simulink model "Test_Hardware"  (R2024a)
settings: Solver=FixedStepAuto  StartTime=0.0  StopTime=inf  FixedStep=0.001  RelTol=1e-3  EnableMultiTasking=on
undefined symbols (not defined in the file or in its folder): g, Jr, k, kp, kv, Lr, mr
libraries: arduinolib x3, arduinosensorlib x2, eeGeneralControl x2
settings Model: ExtModeTrigDuration=2  Creator=Ingy  LastModifiedBy=Ingy
settings SolverCC: AutoInsertRateTranBlk=on
settings OptimizationCC: EnhancedBackFolding=on  PassReuseOutputArgsAs=Individual arguments  ZeroExternalMemoryAtStartup=off  ZeroInternalMemoryAtStartup=off  MaxStackSize=64  OptimizeBlockOrder=speed  DifferentSizesBufferReuse=on  OptimizationCustomize=off  EfficientTunableParamExpr=on
settings DebuggingCC: ParameterTunabilityLossMsg=error
settings HardwareCC: ProdBitPerPointer=32  ProdBitPerSizeT=32  ProdBitPerPtrDiffT=32  ProdLargestAtomicInteger=Long  ProdLargestAtomicFloat=Double  ProdWordSize=32  ProdHWDeviceType=ARM Compatible->ARM Cortex  UseEmbeddedCoderFeatures=off
settings SFSimCC: MATLABDynamicMemAlloc=off
settings RTWCC: Description=Embedded Coder  SystemTargetFile=ert.tlc  HardwareBoard=ESP32-WROOM(Arduino Compatible)  TLCOptions="-aInlineSetEventsForThisBaseRateFcn=TLC_FALSE -aSuppressMultiTaskScheduler=TLC_FALSE  -aRateBasedStepFcn=0"  TemplateMakefile=ert_default_tmf  Toolchain=ESP32  BuildConfiguration=Faster Runs
settings CodeAppCC: ForceParamTrailComments=on  IgnoreCustomStorageClasses=off  OperatorAnnotations=on  SimulinkDataObjDesc=on  SFDataObjDesc=on  InsertBlockDesc=on
settings ERTTargetCC: SupportContinuousTime=on  SupportNonInlinedSFcns=on  SupportVariableSizeSignals=on  ExtModeTransport=3  ExtModeStaticAlloc=on  ExtModeAutomaticAllocSize=off  ExtModeStaticAllocSize=65536  ExtModeMexFile=ext_xcp  ExtModeIntrfLevel=Level2 - Open

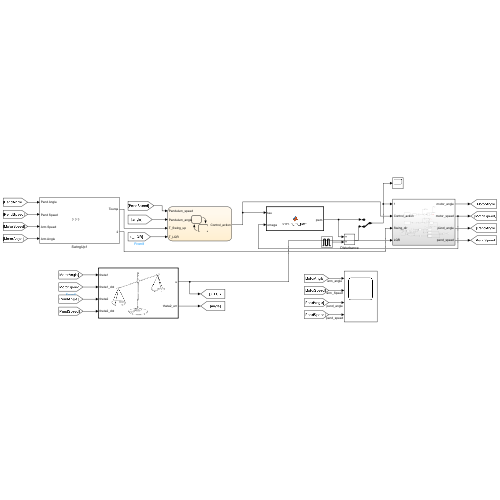
[thumbnail: Simulink's stored preview of the top-level diagram]
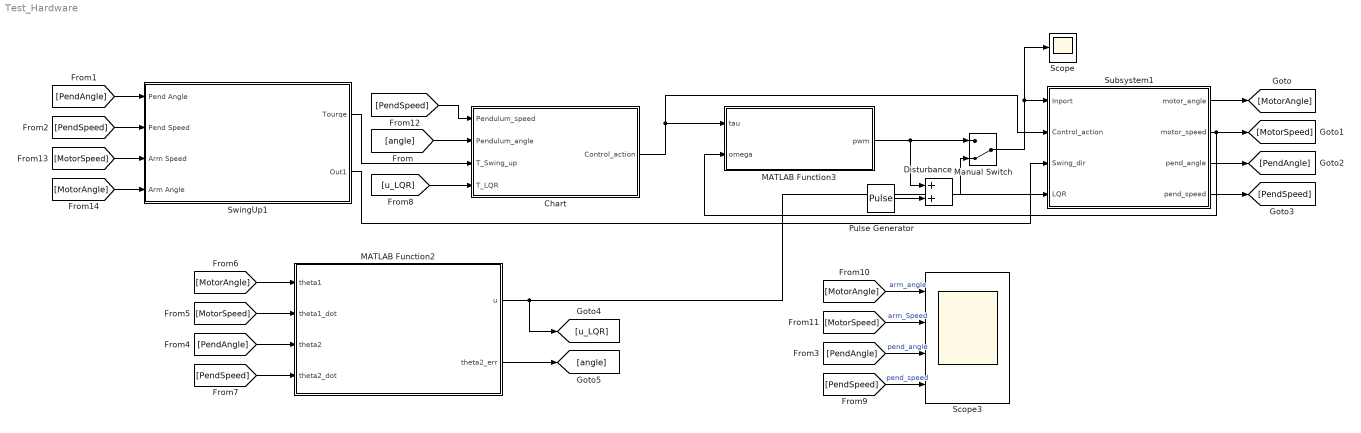
== system Test_Hardware ==
  Chart : Stateflow chart  TreatAsAtomicUnit=on
  Disturbance : Sum
  MATLAB Function2 : MATLAB Function  TreatAsAtomicUnit=on  SystemSampleTime=0.001
  MATLAB Function3 : MATLAB Function  TreatAsAtomicUnit=on
  Manual Switch : ManualSwitch  CurrentSetting=0
  Pulse Generator : DiscretePulseGenerator  PulseType=Time based  Amplitude=90  Period=500  PulseWidth=0.05  PhaseDelay=1
  Scope : Scope
  Scope3 : Scope  NumInputPorts=4
  Subsystem1 : Subsystem
  SwingUp1 : Subsystem
      mask Display: image('download.jpg', [5,5,5,5,100,100]);
  wires:
  [PendAngle] -> SwingUp1/1(Pend Angle)
  Subsystem1/3(pend_angle) -> [PendAngle]
  [PendSpeed] -> Scope3/4  "pend_speed"
  [PendSpeed] -> SwingUp1/2(Pend Speed)
  Subsystem1/1(motor_angle) -> [MotorAngle]
  Subsystem1/4(pend_speed) -> [PendSpeed]
  [MotorAngle] -> Scope3/1  "arm_angle"
  [u_LQR] -> Chart/4(T_LQR)
  [PendAngle] -> Scope3/3  "pend_angle"
  [MotorSpeed] -> Scope3/2  "arm_Speed"
  Manual Switch/1 -> Scope/1, Subsystem1/1(Inport)
  Subsystem1/2(motor_speed) -> MATLAB Function3/2(omega), [MotorSpeed]
  [MotorSpeed] -> SwingUp1/3(Arm Speed)
  [MotorAngle] -> SwingUp1/4(Arm Angle)
  [MotorAngle] -> MATLAB Function2/1(theta1)
  [MotorSpeed] -> MATLAB Function2/2(theta1_dot)
  [PendAngle] -> MATLAB Function2/3(theta2)
  [PendSpeed] -> MATLAB Function2/4(theta2_dot)
  SwingUp1/2(Out1) -> Subsystem1/3(Swing_dir)
  MATLAB Function2/1(u) -> [u_LQR], Subsystem1/4(LQR)
  SwingUp1/1(Tourqe) -> Chart/3(T_Swing_up)
  Chart/1(Control_action) -> Subsystem1/2(Control_action), MATLAB Function3/1(tau)
  MATLAB Function2/2(theta2_err) -> [angle]
  [angle] -> Chart/2(Pendulum_angle)
  [PendSpeed] -> Chart/1(Pendulum_speed)
  Disturbance/1 -> Manual Switch/2
  Pulse Generator/1 -> Disturbance/2
  MATLAB Function3/1(pwm) -> Manual Switch/1, Disturbance/1

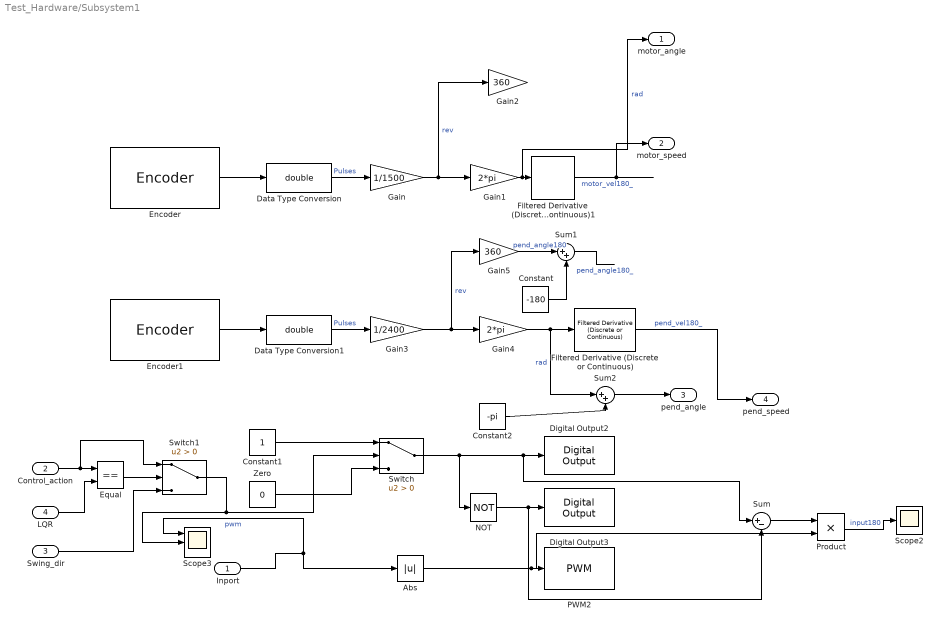
== system Test_Hardware/Subsystem1 ==
  Inport : Inport
  Control_action : Inport  Port=2
  Swing_dir : Inport  Port=3
  LQR : Inport  Port=4
  Abs : Abs  SaturateOnIntegerOverflow=off
  Constant : Constant  Value=-180
  Constant1 : Constant
  Constant2 : Constant  Value=-pi
  Data Type Conversion : DataTypeConversion  OutDataTypeStr=double  SaturateOnIntegerOverflow=off  RndMeth=Floor
  Data Type Conversion1 : DataTypeConversion  OutDataTypeStr=double  SaturateOnIntegerOverflow=off  RndMeth=Floor
  Digital Output2 : arduinolib/Digital Output  pinNumber=23  Direction=output  blockPlatform=arduino
  Digital Output3 : arduinolib/Digital Output  pinNumber=22  Direction=output  blockPlatform=arduino
  Encoder : arduinosensorlib/Encoder  InputA=25  InputB=26  Mode=No reset  SampleTime=-1
  Encoder1 : arduinosensorlib/Encoder  InputA=19  InputB=18  Mode=No reset  SampleTime=-1
  Equal : RelationalOperator  Operator===  OutDataTypeStr=boolean  RndMeth=Simplest  InputSameDT=off
  Filtered Derivative (Discrete or Continuous) : eeGeneralControl/Filtered Derivative (Discrete or Continuous)  K=1  T=0.07  B=inf  A=-inf  minRatio=10  init_option=Inherited from block input  x0=0  Ts=-1
      settings: LibrarySourceBlock=|
      | ee_sl_lib/General Control/Filtered Derivative
      | (Discrete or Continuous)
  Filtered Derivative (Discrete or Continuous)1 : eeGeneralControl/Filtered Derivative (Discrete or Continuous)  K=1  T=0.07  B=inf  A=-inf  minRatio=10  init_option=Inherited from block input  x0=0  Ts=-1
      settings: LibrarySourceBlock=|
      | ee_sl_lib/General Control/Filtered Derivative
      | (Discrete or Continuous)
  Gain : Gain  Gain=1/1500
  Gain1 : Gain  Gain=2*pi
  Gain2 : Gain  Gain=360
  Gain3 : Gain  Gain=1/2400
  Gain4 : Gain  Gain=2*pi
  Gain5 : Gain  Gain=360
  NOT : Logic  Operator=NOT  IconShape=distinctive  AllPortsSameDT=off  OutDataTypeStr=boolean
  PWM2 : arduinolib/PWM  pinNumber=21  frequencyType=Default  desiredFrequency=800  achievableFrequency=800
  Product : Product
  Scope2 : Scope
  Scope3 : Scope  NumInputPorts=3
  Sum : Sum  Inputs=|+-
  Sum1 : Sum  Inputs=|++
  Sum2 : Sum  Inputs=|++
  Switch : Switch  Criteria=u2 > Threshold  SaturateOnIntegerOverflow=off  InputSameDT=off
  Switch1 : Switch  Criteria=u2 > Threshold  SaturateOnIntegerOverflow=off  InputSameDT=off
  Zero : Constant  Value=0  OutDataTypeStr=Inherit: Inherit via back propagation
  motor_angle : Outport
  motor_speed : Outport  Port=2
  pend_angle : Outport  Port=3
  pend_speed : Outport  Port=4
  wires:
  Sum1/1 -> ?  "pend_angle180_"
  Gain5/1 -> Sum1/1  "pend_angle180"
  Filtered Derivative (Discrete or Continuous)1/1 -> motor_speed/1  "motor_vel180_"
  Data Type Conversion/1 -> Gain/1  "Pulses"
  Gain/1 -> Gain2/1, Gain1/1  "rev"
  Filtered Derivative (Discrete or Continuous)/1 -> pend_speed/1  "pend_vel180_"
  Gain4/1 -> Sum2/1, Filtered Derivative (Discrete or Continuous)/1  "rad"
  Data Type Conversion1/1 -> Gain3/1  "Pulses"
  Gain3/1 -> Gain5/1, Gain4/1  "rev"
  Constant/1 -> Sum1/2
  Encoder/1 -> Data Type Conversion/1
  Gain1/1 -> motor_angle/1, Filtered Derivative (Discrete or Continuous)1/1  "rad"
  Encoder1/1 -> Data Type Conversion1/1
  Inport/1 -> Abs/1, Scope3/1  "pwm"
  Constant1/1 -> Switch/1
  Zero/1 -> Switch/3
  NOT/1 -> Sum/2, Digital Output3/1
  Abs/1 -> Product/2, PWM2/1
  Product/1 -> Scope2/1  "input180"
  Sum/1 -> Product/1
  Switch/1 -> NOT/1, Sum/1, Digital Output2/1
  Constant2/1 -> Sum2/2
  Sum2/1 -> pend_angle/1
  LQR/1 -> Equal/2
  Swing_dir/1 -> Switch1/3
  Switch1/1 -> Scope3/2, Switch/2
  Control_action/1 -> Switch1/1, Equal/1
  Equal/1 -> Switch1/2

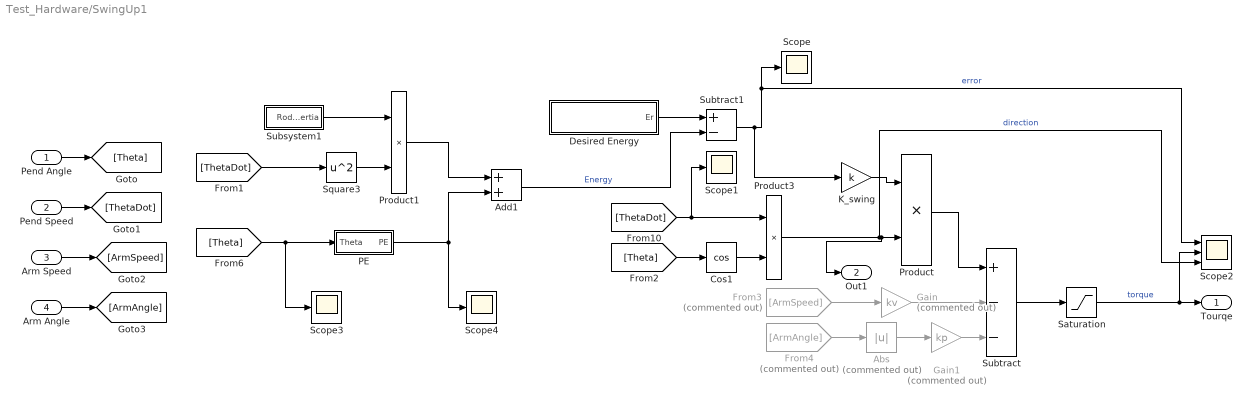
== system Test_Hardware/SwingUp1 ==
  Pend Angle : Inport
  Pend Speed : Inport  Port=2
  Arm Speed : Inport  Port=3
  Arm Angle : Inport  Port=4
  Abs : Abs  Commented=on  SaturateOnIntegerOverflow=off
  Add1 : Sum
  Cos1 : Trigonometry  Operator=cos
  Desired Energy : Subsystem
  From3 : From  Commented=on  GotoTag=ArmSpeed
  From4 : From  Commented=on  GotoTag=ArmAngle
  Gain : Gain  Commented=on  Gain=kv
  Gain1 : Gain  Commented=on  Gain=kp
  K_swing : Gain  Gain=k
  PE : Subsystem
  Product : Product
  Product1 : Product
  Product3 : Product
  Saturation : Saturate  UpperLimit=3  LowerLimit=-3
  Scope{,1,3..4} (4 alike) : Scope
  Scope2 : Scope  NumInputPorts=3
  Square3 : Math  Operator=square
  Subsystem1 : Subsystem
  Subtract : Sum  Inputs=+--
  Subtract1 : Sum  Inputs=+-
  Tourqe : Outport
  Out1 : Outport  Port=2
  wires:
  Pend Angle/1 -> [Theta]
  Pend Speed/1 -> [ThetaDot]
  Subsystem1/1(RodInertia) -> Product1/1
  Product1/1 -> Add1/1
  PE/1(PE) -> Scope4/1, Add1/2
  K_swing/1 -> Product/1
  Desired Energy/1(Er) -> Subtract1/1
  Subtract1/1 -> Scope2/1, Scope/1, K_swing/1  "error"
  [Theta] -> Cos1/1
  Cos1/1 -> Product3/2
  Add1/1 -> Subtract1/2  "Energy"
  [ThetaDot] -> Square3/1
  Square3/1 -> Product1/2
  [ThetaDot] -> Product3/1, Scope1/1
  Saturation/1 -> Scope2/2, Tourqe/1  "torque"
  Arm Speed/1 -> [ArmSpeed]
  Gain/1 -> Subtract/2
  Product/1 -> Subtract/1
  Subtract/1 -> Saturation/1
  [Theta] -> Scope3/1, PE/1(Theta)
  Arm Angle/1 -> [ArmAngle]
  Gain1/1 -> Subtract/3
  Product3/1 -> Out1/1, Product/2, Scope2/3  "direction"
  From3/1 -> Gain/1
  From4/1 -> Abs/1
  Abs/1 -> Gain1/1

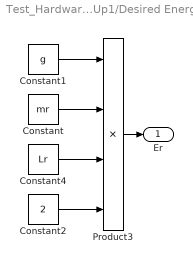
== system Test_Hardware/SwingUp1/Desired Energy ==
  Constant : Constant  Value=mr
  Constant1 : Constant  Value=g
  Constant2 : Constant  Value=2
  Constant4 : Constant  Value=Lr
  Product3 : Product  Inputs=4
  Er : Outport
  wires:
  Constant1/1 -> Product3/1
  Constant/1 -> Product3/2
  Constant4/1 -> Product3/3
  Product3/1 -> Er/1
  Constant2/1 -> Product3/4

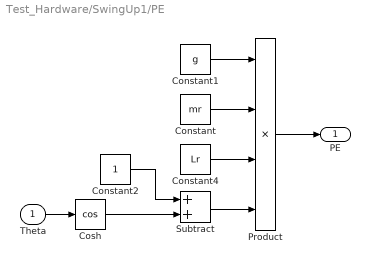
== system Test_Hardware/SwingUp1/PE ==
  Theta : Inport
  Constant : Constant  Value=mr
  Constant1 : Constant  Value=g
  Constant2 : Constant
  Constant4 : Constant  Value=Lr
  Cosh : Trigonometry  Operator=cos
  Product : Product  Inputs=4
  Subtract : Sum
  PE : Outport
  wires:
  Constant1/1 -> Product/1
  Constant/1 -> Product/2
  Constant4/1 -> Product/3
  Theta/1 -> Cosh/1
  Product/1 -> PE/1
  Subtract/1 -> Product/4
  Constant2/1 -> Subtract/1
  Cosh/1 -> Subtract/2

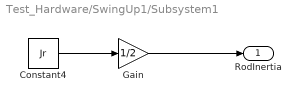
== system Test_Hardware/SwingUp1/Subsystem1 ==
  Constant4 : Constant  Value=Jr
  Gain : Gain  Gain=1/2
  RodInertia : Outport
  wires:
  Constant4/1 -> Gain/1
  Gain/1 -> RodInertia/1

== stateflow chart Test_Hardware/Chart ==
  settings: updateMethod=DISCRETE  sampleTime=0.001
  state Swing_mode
    entry:
    Control_action = T_Swing_up
    during:
    Control_action = T_Swing_up
  state LQR_mode
    entry:
    Control_action = T_LQR
    during:
    Control_action = T_LQR
  (default) -> Swing_mode
  Swing_mode -> LQR_mode : [abs(Pendulum_angle)<=15*pi/180 && abs(Pendulum_speed)<=3.5]
  LQR_mode -> Swing_mode : [abs(Pendulum_angle)>=15*pi/180]
  data: Pendulum_speed input; Pendulum_angle input; Control_action output; T_Swing_up input; T_LQR input

== matlab function Test_Hardware/MATLAB Function2 ==
  settings: updateMethod=DISCRETE
  data: theta1 input; theta1_dot input; theta2 input; theta2_dot input; u output; theta2_err output
function [u, theta2_err]= LQR_controller(theta1, theta1_dot, theta2, theta2_dot)
% LQR stabilizer for Furuta pendulum
% Upright at theta2 = 0 (or 2*pi)
% No swing-up, no memory

% LQR gain
K_ = [-0.316227766016342,-0.203276132698185,5.614675633123943,0.557548956161459];
% K_ = [-0.0100000000000004, -0.0857445820450138, 1.58797510295829, 0.147807220044965];

% Step 1: wrap to [0, 2*pi) to avoid huge numbers
theta2_wrapped = mod(theta2, 2*pi);

% Step 2: compute shortest distance to upright (0)
theta2_err = atan2(sin(theta2_wrapped), cos(theta2_wrapped));

% State vector
x = [theta1;
     theta1_dot;
     theta2_err;
     theta2_dot];

% LQR control
if(abs(theta2_err)<=20*pi/180)
    u = -K_ * x;
else
    u = 0;
end

end

== matlab function Test_Hardware/MATLAB Function3 ==
  data: tau input; pwm output; omega input
function pwm = torque_to_pwm(tau, omega)

% === Motor parameters (estimated) ===
Kt = 12*60/(2*pi*250);       % Nm/A
Ke = Kt;       % V/(rad/s)
R  =  5.8466;        % Ohms
Vmax = 12;       % Supply voltage

% === Torque → Voltage ===
V = (tau / Kt) * R + Ke * omega;

% === Voltage → PWM ===
pwm = 255 * V / Vmax;

% === Saturation ===
pwm = max(min(pwm,210),-210);

end
